simulink model "sim_pid"  (R2023b)
settings: Solver=FixedStepAuto  StartTime=0.0  StopTime=100  FixedStep=0.0001  RelTol=1e-3
values from neighbouring files (symbols this model uses):
  denom_obj = [ a01^3, 3*(a01^2)*a00, 3*a01*a00^2, a00^3]    [regulator_pid.m]
  denom_pid_derivative = [ 0.0001, 1]    [regulator_pid.m]
  denom_pid_gain = [ 0, 1]    [regulator_pid.m]
  denom_pid_integral = [ Ti, 0]    [regulator_pid.m]
  final_value = 1    [regulator_pid.m]
  initial_value = 0    [regulator_pid.m]
  nom_obj = [ 0, 0, 0, 1 ]    [regulator_pid.m]
  nom_pid_derivative = [ Td, 0]    [regulator_pid.m]
  nom_pid_gain = [ 0, K ]    [regulator_pid.m]
  nom_pid_integral = [ 0, 1]    [regulator_pid.m]
  step_time = 0    [regulator_pid.m]
settings Model: Creator=tomasz  LastModifiedBy=tomasz

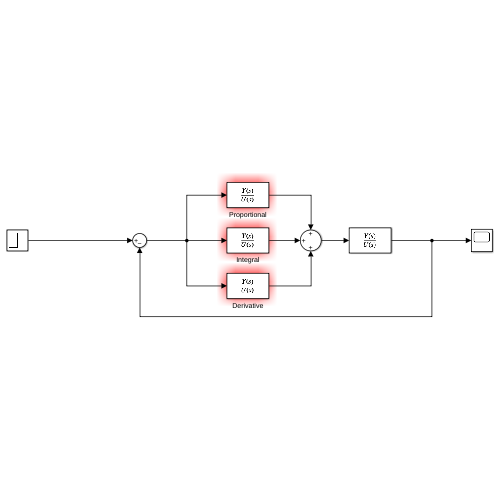
[thumbnail: Simulink's stored preview of the top-level diagram]
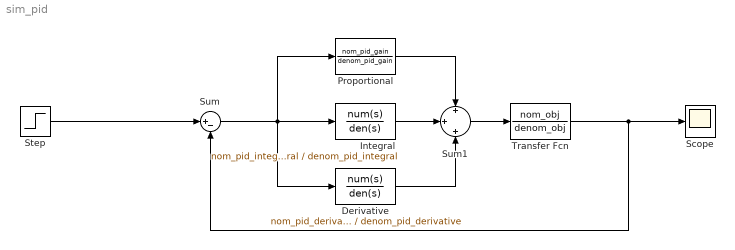
== system sim_pid ==
  Derivative : TransferFcn  Numerator=nom_pid_derivative  Denominator=denom_pid_derivative
  Integral : TransferFcn  Numerator=nom_pid_integral  Denominator=denom_pid_integral
  Proportional : TransferFcn  Numerator=nom_pid_gain  Denominator=denom_pid_gain
  Scope : Scope
  Step : Step  Time=step_time  Before=initial_value  After=final_value  SampleTime=0
  Sum : Sum  Inputs=|+-
  Sum1 : Sum  Inputs=+|+|+
  Transfer Fcn : TransferFcn  Numerator=nom_obj  Denominator=denom_obj
  wires:
  Step/1 -> Sum/1
  Sum/1 -> Derivative/1, Proportional/1, Integral/1
  Transfer Fcn/1 -> Sum/2, Scope/1
  Integral/1 -> Sum1/2
  Proportional/1 -> Sum1/1
  Derivative/1 -> Sum1/3
  Sum1/1 -> Transfer Fcn/1
